simulink model "STR"  (R2023a)
settings: Solver=VariableStepAuto  StartTime=0.0  StopTime=10.0  RelTol=1e-3
settings Model: Creator=Mmoha  LastModifiedBy=Mmoha

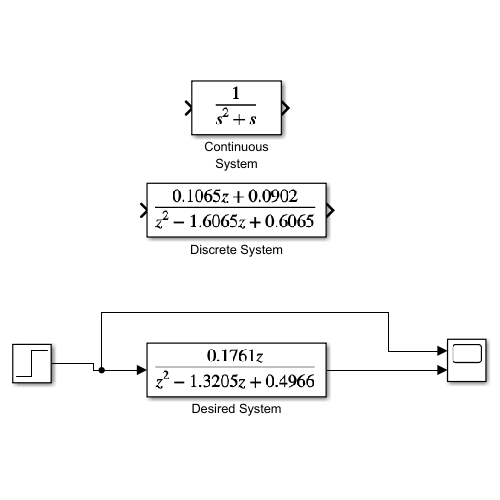
[thumbnail: Simulink's stored preview of the top-level diagram]
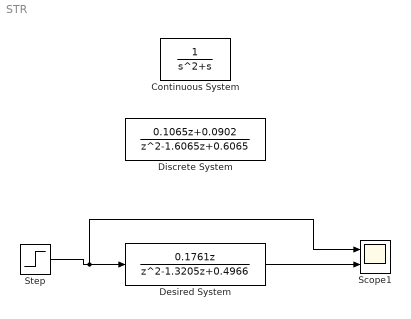
== system STR ==
  Continuous System : TransferFcn  Numerator=[0 0 1]  Denominator=[1 1 0]
  Desired System : DiscreteTransferFcn  Numerator=[0.1761 0]  Denominator=[1 -1.3205 0.4966]  SampleTime=0.5
  Discrete System : DiscreteTransferFcn  Numerator=[0 0.1065 0.0902]  Denominator=[1 -1.6065 0.6065]  SampleTime=0.5
  Scope1 : Scope  NumInputPorts=2
  Step : Step  SampleTime=0
  wires:
  Step/1 -> Scope1/1, Desired System/1
  Desired System/1 -> Scope1/2
